simulink model "Majority_Voter"  (R2018b)
settings: Solver=VariableStepAuto  StartTime=0.0  StopTime=10.0  RelTol=1e-3
settings Model: Creator=jayakumarav  LastModifiedBy=jayakumarav

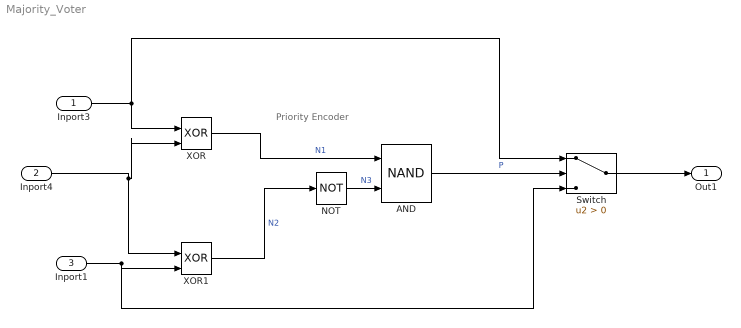
== system Majority_Voter ==
  note: Priority Encoder
  Inport3 : Inport
  Inport4 : Inport  Port=2
  Inport1 : Inport  Port=3
  AND : Logic  Operator=NAND  IconShape=distinctive  AllPortsSameDT=off  OutDataTypeStr=boolean
  NOT : Logic  Operator=NOT  IconShape=distinctive  AllPortsSameDT=off  OutDataTypeStr=boolean
  Switch : Switch  Criteria=u2 > Threshold
  XOR : Logic  Operator=XOR  IconShape=distinctive  AllPortsSameDT=off  OutDataTypeStr=boolean
  XOR1 : Logic  Operator=XOR  IconShape=distinctive  AllPortsSameDT=off  OutDataTypeStr=boolean
  Out1 : Outport
  wires:
  Inport3/1 -> Switch/1, XOR/1
  Inport4/1 -> XOR1/1, XOR/2
  Inport1/1 -> Switch/3, XOR1/2
  NOT/1 -> AND/2  "N3"
  XOR1/1 -> NOT/1  "N2"
  XOR/1 -> AND/1  "N1"
  AND/1 -> Switch/2  "P"
  Switch/1 -> Out1/1
